simulink model "Lecture14b_MotorControlv5_FeedForward"  (R2022a)
settings: Solver=ode4  StartTime=0.0  StopTime=0.4  FixedStep=0.0001  RelTol=1e-3
undefined symbols (not defined in the file): b, J, K0, K1, K2, Ke, Kt, L, R
libraries: slpidlib x1
settings Model: Creator=hwang  LastModifiedBy=hwang
settings SolverCC: EnableFixedStepZeroCrossing=on

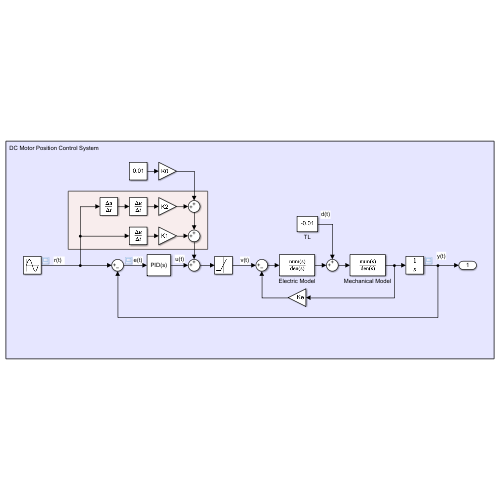
[thumbnail: Simulink's stored preview of the top-level diagram]
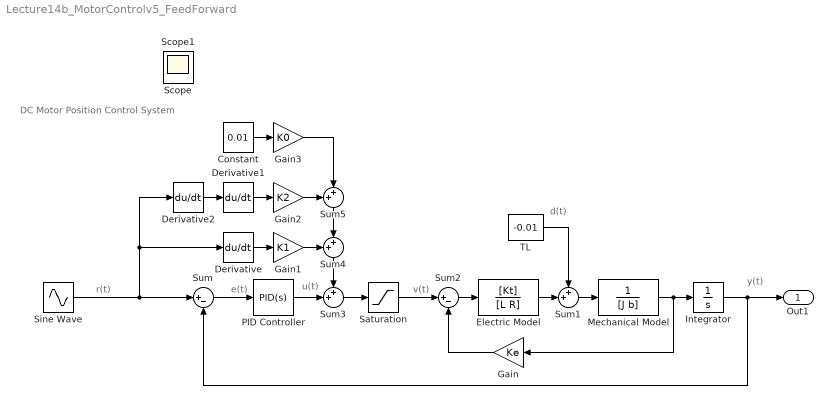
== system Lecture14b_MotorControlv5_FeedForward ==
  note: v(t)
  note: d(t)
  note: DC Motor Position Control System
  note: e(t)
  note: u(t)
  note: r(t)
  note: y(t)
  Constant : Constant  Value=0.01
  Derivative : Derivative
  Derivative1 : Derivative
  Derivative2 : Derivative
  Electric Model : TransferFcn  Numerator=[Kt]  Denominator=[L R]
  Gain : Gain  Gain=Ke
  Gain1 : Gain  Gain=K1
  Gain2 : Gain  Gain=K2
  Gain3 : Gain  Gain=K0
  Integrator : Integrator
  Mechanical Model : TransferFcn  Denominator=[J b]
  PID Controller : slpidlib/PID Controller  Controller=PID  Form=Parallel  TimeDomain=Continuous-time  UseExternalTs=off  SampleTime=-1  IntegratorMethod=Forward Euler  FilterMethod=Forward Euler  ControllerParametersSource=internal  P=20  I=400  UseKiTs=off  D=0.1  N=1000  UseFilter=on  TunerSelectOption=Transfer Function Based (PID Tuner App)  InitialConditionSource=internal  InitialConditionForIntegrator=0  InitialConditionForFilter=0  DifferentiatorICPrevScaledInput=0  ExternalReset=none  TrackingMode=off  Kt=1  LimitOutput=off  SatLimitsSource=internal  UpperSaturationLimit=inf  LowerSaturationLimit=-inf  LinearizeAsGain=on  AntiWindupMode=none  Kb=1  POutMin=[]  POutMax=[]  IOutMin=[]  IOutMax=[]  DOutMin=[]  DOutMax=[]  NOutMin=[]  NOutMax=[]  SumOutMin=[]  SumOutMax=[]  SaturationOutMin=[]  SaturationOutMax=[]  PParamMin=[]  PParamMax=[]  IParamMin=[]  IParamMax=[]  DParamMin=[]  DParamMax=[]  NParamMin=[]  NParamMax=[]  KbParamMin=[]  KbParamMax=[]  KtParamMin=[]  KtParamMax=[]  KbOutMin=[]  KbOutMax=[]  KtOutMin=[]  KtOutMax=[]  IntegratorOutMin=[]  IntegratorOutMax=[]  FilterOutMin=[]  FilterOutMax=[]  SumI1OutMin=[]  SumI1OutMax=[]  SumI2OutMin=[]  SumI2OutMax=[]  SumI3OutMin=[]  SumI3OutMax=[]  SumI4OutMin=[]  SumI4OutMax=[]  SumDOutMin=[]  SumDOutMax=[]  DifferentiatorOutMin=[]  DifferentiatorOutMax=[]  FilterDiffOutCoefMin=[]  FilterDiffOutCoefMax=[]  ReciprocalOutMin=[]  ReciprocalOutMax=[]  SumDenOutMin=[]  SumDenOutMax=[]  SumNumOutMin=[]  SumNumOutMax=[]  DivideOutMin=[]  DivideOutMax=[]  UdiffTsProdOutMin=[]  UdiffTsProdOutMax=[]  NTsProdOutMin=[]  NTsProdOutMax=[]  UintegralTsProdOutMin=[]  UintegralTsProdOutMax=[]  UngainTsProdOutMin=[]  UngainTsProdOutMax=[]  IntegratorContinuousStateAttributes=''  IntegratorStateMustResolveToSignalObject=off  IntegratorRTWStateStorageClass=Auto  FilterContinuousStateAttributes=''  FilterStateMustResolveToSignalObject=off  FilterRTWStateStorageClass=Auto  ParallelPVariant=InternalParameters  IdealPVariant=Disabled  IVariant=InternalParameters  DVariant=InternalParameters  IntegratorVariant=Continuous  SatVariant=Disabled  AWVariant=Passthrough  PCopyVariant=Disabled  TRVariant=Disabled  FdbkBlocksVariant=Forward  IdealPFdbkVariant=Disabled  SatFdbkVariant=Disabled  DerivativeFilterVariant=ContFilter  NVariant=InternalParameters  NCopyVariant=Disabled  FilterICVariant=InternalICsFilter  IntegratorICVariant=InternalICs  ExternalResetVariant=Disabled  TRSumVariant=Passthrough  SumFdbkVariant=Disabled  SumVariant=Sum_PID  TsampFilterVariant=InternalTs  TsampNgainVariant=Passthrough  TsampIntegralVariant=Passthrough  ExternalSaturationOutDataTypeStr=Inherit: Same as second input  aMode=0
  Saturation : Saturate  UpperLimit=24  LowerLimit=-24
  Sine Wave : Sin  Bias=1  Frequency=(2*3.141592)*5  Phase=-3.141592/2  SampleTime=0
  Sum : Sum  Inputs=|+-
  Sum{1,3..5} (4 alike) : Sum  Inputs=++|
  Sum2 : Sum  Inputs=|+-
  TL : Constant  Value=-0.01
  Out1 : Outport
  Scope : Scope
  Scope1 : Scope
  wires:
  Sum/1 -> PID Controller/1
  PID Controller/1 -> Sum3/2
  Mechanical Model/1 -> Integrator/1, Gain/1
  Electric Model/1 -> Sum1/2
  Sum1/1 -> Mechanical Model/1
  TL/1 -> Sum1/1
  Integrator/1 -> Out1/1, Sum/2
  Sum2/1 -> Electric Model/1
  Gain/1 -> Sum2/2
  Saturation/1 -> Sum2/1
  Sine Wave/1 -> Derivative/1, Derivative2/1, Sum/1
  Sum3/1 -> Saturation/1
  Derivative/1 -> Gain1/1
  Derivative2/1 -> Derivative1/1
  Derivative1/1 -> Gain2/1
  Gain1/1 -> Sum4/1
  Gain2/1 -> Sum5/1
  Sum5/1 -> Sum4/2
  Sum4/1 -> Sum3/1
  Constant/1 -> Gain3/1
  Gain3/1 -> Sum5/2
